simulink model "task32"  (R2024a)
settings: Solver=VariableStepAuto  StartTime=0.0  StopTime=10.0  MaxStep=0.01  RelTol=1e-3
undefined symbols (not defined in the file): A, B, Bf, C, D, Df, Gamma, Gamma_f, Gamma_ff, Gamma_g, K, Kf, Kg, Q, Qff, wf0, wf_bar, wg0, wg0_bar, x0, Y, Yf, Yff, Yg
settings Model: Creator=sizgr  LastModifiedBy=sizgr

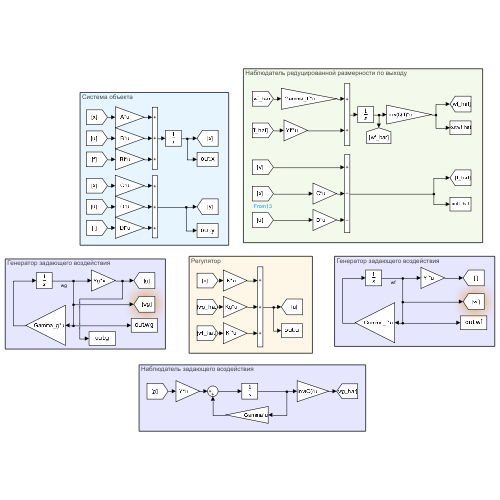
[thumbnail: Simulink's stored preview of the top-level diagram]
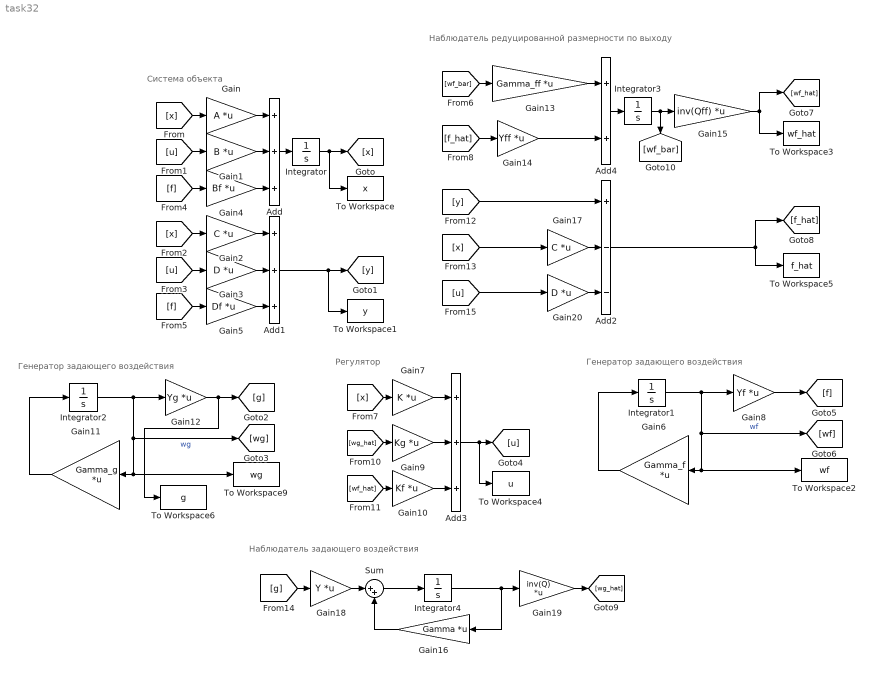
== system task32 ==
  note: Наблюдатель задающего воздействия
  note: Наблюдатель редуцированной размерности по выходу
  note: Генератор задающего воздействия
  note: Регулятор
  note: Система объекта
  note: Генератор задающего воздействия
  Add : Sum  Inputs=+++
  Add1 : Sum  Inputs=+++
  Add2 : Sum  Inputs=+--
  Add3 : Sum  Inputs=+++
  Add4 : Sum
  Gain : Gain  Gain=A  Multiplication=Matrix(K*u)
  Gain1 : Gain  Gain=B  Multiplication=Matrix(K*u)
  Gain10 : Gain  Gain=Kf  Multiplication=Matrix(K*u)
  Gain11 : Gain  Gain=Gamma_g  Multiplication=Matrix(K*u)
  Gain12 : Gain  Gain=Yg  Multiplication=Matrix(K*u)
  Gain13 : Gain  Gain=Gamma_ff  Multiplication=Matrix(K*u)
  Gain14 : Gain  Gain=Yff  Multiplication=Matrix(K*u)
  Gain15 : Gain  Gain=inv(Qff)  Multiplication=Matrix(K*u)
  Gain16 : Gain  Gain=Gamma  Multiplication=Matrix(K*u)
  Gain17 : Gain  Gain=C  Multiplication=Matrix(K*u)
  Gain18 : Gain  Gain=Y  Multiplication=Matrix(K*u)
  Gain19 : Gain  Gain=inv(Q)  Multiplication=Matrix(K*u)
  Gain2 : Gain  Gain=C  Multiplication=Matrix(K*u)
  Gain20 : Gain  Gain=D  Multiplication=Matrix(K*u)
  Gain3 : Gain  Gain=D  Multiplication=Matrix(K*u)
  Gain4 : Gain  Gain=Bf  Multiplication=Matrix(K*u)
  Gain5 : Gain  Gain=Df  Multiplication=Matrix(K*u)
  Gain6 : Gain  Gain=Gamma_f  Multiplication=Matrix(K*u)
  Gain7 : Gain  Gain=K  Multiplication=Matrix(K*u)
  Gain8 : Gain  Gain=Yf  Multiplication=Matrix(K*u)
  Gain9 : Gain  Gain=Kg  Multiplication=Matrix(K*u)
  Integrator : Integrator  InitialCondition=x0
  Integrator1 : Integrator  InitialCondition=wf0
  Integrator2 : Integrator  InitialCondition=wg0
  Integrator3 : Integrator  InitialCondition=wf_bar
  Integrator4 : Integrator  InitialCondition=wg0_bar
  Sum : Sum  Inputs=|++
  To Workspace : ToWorkspace  VariableName=x  SaveFormat=Timeseries  SampleTime=-1
  To Workspace1 : ToWorkspace  VariableName=y  SaveFormat=Timeseries  SampleTime=-1
  To Workspace2 : ToWorkspace  VariableName=wf  SaveFormat=Timeseries  SampleTime=-1
  To Workspace3 : ToWorkspace  VariableName=wf_hat  SaveFormat=Timeseries  SampleTime=-1
  To Workspace4 : ToWorkspace  VariableName=u  SaveFormat=Timeseries  SampleTime=-1
  To Workspace5 : ToWorkspace  VariableName=f_hat  SaveFormat=Timeseries  SampleTime=-1
  To Workspace6 : ToWorkspace  VariableName=g  SaveFormat=Timeseries  SampleTime=-1
  To Workspace9 : ToWorkspace  VariableName=wg  SaveFormat=Timeseries  SampleTime=-1
  wires:
  Add/1 -> Integrator/1
  Gain/1 -> Add/1
  Gain1/1 -> Add/2
  Integrator/1 -> To Workspace/1, [x]
  [x] -> Gain/1
  [u] -> Gain1/1
  Gain2/1 -> Add1/1
  [u] -> Gain3/1
  Add1/1 -> To Workspace1/1, [y]
  [x] -> Gain2/1
  Gain3/1 -> Add1/2
  Add3/1 -> To Workspace4/1, [u]
  Gain7/1 -> Add3/1
  Gain9/1 -> Add3/2
  Gain10/1 -> Add3/3
  [x] -> Gain7/1
  [wg_hat] -> Gain9/1
  [wf_hat] -> Gain10/1
  Integrator2/1 -> Gain12/1, To Workspace9/1, Gain11/1, [wg]  "wg"
  Gain11/1 -> Integrator2/1
  Gain12/1 -> To Workspace6/1, [g]
  [f] -> Gain4/1
  Gain4/1 -> Add/3
  [f] -> Gain5/1
  Gain5/1 -> Add1/3
  Gain8/1 -> [f]
  Integrator1/1 -> Gain8/1, To Workspace2/1, Gain6/1, [wf]  "wf"
  Gain6/1 -> Integrator1/1
  Add4/1 -> Integrator3/1
  [wf_bar] -> Gain13/1
  [f_hat] -> Gain14/1
  Gain13/1 -> Add4/1
  Gain14/1 -> Add4/2
  [x] -> Gain17/1
  Add2/1 -> [f_hat], To Workspace5/1
  [y] -> Add2/1
  Gain17/1 -> Add2/2
  Integrator4/1 -> Gain19/1, Gain16/1
  Sum/1 -> Integrator4/1
  Gain16/1 -> Sum/2
  Gain18/1 -> Sum/1
  [g] -> Gain18/1
  Gain19/1 -> [wg_hat]
  [u] -> Gain20/1
  Gain20/1 -> Add2/3
  Integrator3/1 -> Gain15/1, [wf_bar]
  Gain15/1 -> To Workspace3/1, [wf_hat]
